simulink model "Assignment_2_RateAdaptive"  (R2020a)
settings: Solver=FixedStepAuto  StartTime=0.0  StopTime=10.0  FixedStep=1e-3  RelTol=1e-3  EnableMultiTasking=on
undefined symbols (not defined in the file): D0, D1, D10, D11, D12, D13, D2, D3, D4, D5, D6, D7, D8, D9, PTA0, PTA1, PTA2, PTB23, PTB9, PTC16, PTC17, PTC2, PTC3, PTC4, PTD0, PTD1, PTD2, PTD3
libraries: frdmk64flib x18, dspstat3 x1
settings Model: ExtModeTrigDuration=5  Creator=School  LastModifiedBy=logan_duui82v
settings OptimizationCC: EnhancedBackFolding=on  PassReuseOutputArgsAs=Individual arguments  ZeroExternalMemoryAtStartup=off  ZeroInternalMemoryAtStartup=off  MaxStackSize=64  OptimizeBlockOrder=speed  DifferentSizesBufferReuse=on  OptimizationCustomize=off  EfficientTunableParamExpr=on
settings DebuggingCC: ParameterTunabilityLossMsg=error
settings HardwareCC: ProdBitPerPointer=32  ProdBitPerSizeT=32  ProdBitPerPtrDiffT=32  ProdLargestAtomicInteger=Long  ProdLargestAtomicFloat=Double  ProdWordSize=32  ProdHWDeviceType=ARM Compatible->ARM Cortex
settings SFSimCC: MATLABDynamicMemAlloc=off
settings RTWCC: SystemTargetFile=ert.tlc  HardwareBoard=NXP FRDM-K64F  TemplateMakefile=ert_default_tmf  Toolchain=GNU Tools for ARM Embedded Processors
settings CodeAppCC: ForceParamTrailComments=on  IgnoreCustomStorageClasses=off  OperatorAnnotations=on  SimulinkDataObjDesc=on  SFDataObjDesc=on  InsertBlockDesc=on

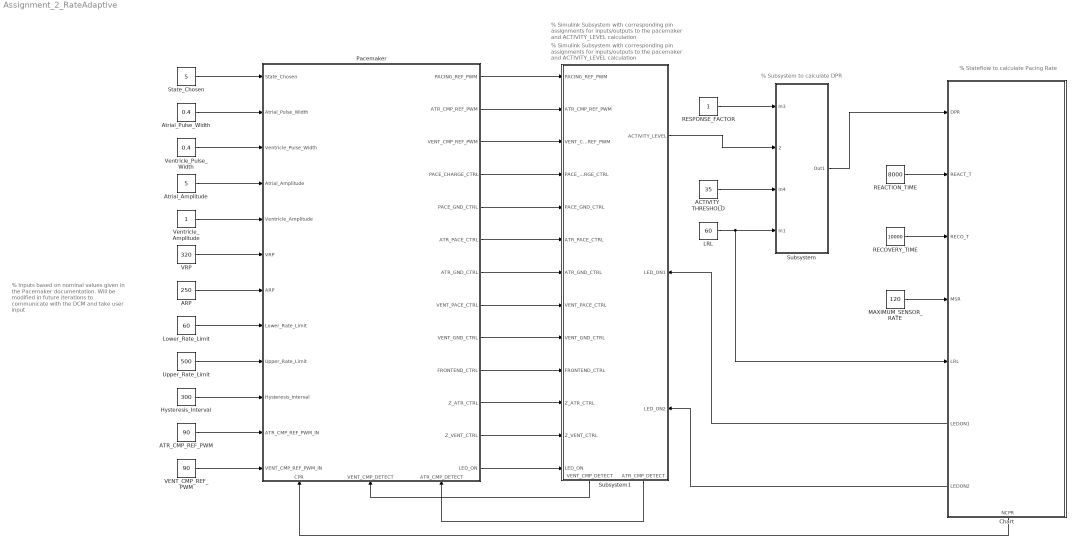
== system Assignment_2_RateAdaptive ==
  note: % Stateflow to calculate Pacing Rate
  note: % Inputs based on nominal values
      | given in the Pacemaker documentation.
      | Will be modified in future iterations to
      | communicate with the DCM and take
      | user input
  note: % Simulink Subsystem with corresponding pin
      | assignments for inputs/outputs to the pacemaker
      | and ACTIVITY_LEVEL calculation
  note: % Subsystem to calculate DPR
  note: % Simulink Subsystem with corresponding pin
      | assignments for inputs/outputs to the pacemaker
      | and ACTIVITY_LEVEL calculation
  ACTIVITY_THRESHOLD : Constant  Value=35
  ARP : Constant  Value=250
  ATR_CMP_REF_PWM : Constant  Value=90
  Atrial_Amplitude : Constant  Value=5  OutDataTypeStr=double
  Atrial_Pulse_Width : Constant  Value=0.4  OutDataTypeStr=int32
  Chart : Stateflow chart  TreatAsAtomicUnit=on
      settings: PortSchema="{\"entries\":[{\"content\":{\"sides\":[{\"content\":{\"connectorIds\":[\"In5\",\"In1\",\"In2\",\"In3\",\"In4\",\"Out2\",\"Out3\"]},\"type\":\"ConnectorPlacement.EquallySpacedRectSide\",\"uuid\":\"cb49ebd1-b2c7-4a1e-b062-18a1bf51e97f\"},{\"content\":{\"connectorIds\":[],\"side\":\"RIGHT\"},\"type\":\"ConnectorPlacement.EquallySpacedRectSide\",\"uuid\":\"35cf40a1-f02a-4965-9a15-2487395dd71b\"},{\"content\":{\"connectorIds\":[],\"side\":\"TOP\"},\"type\":\"ConnectorPlacement.EquallySpacedRectSide\",\"uuid\":\"8cf7664f-bebd-444c-a693-a1ee33fcaf3f\"},{\"content\":{\"connectorIds\":[\"Out1\"],\"side\":\"BOTTOM\"},\"type\":\"ConnectorPlacement.EquallySpacedRectSide\",\"uuid\":\"96b9c03b-a83e-462b-a12d-192e0bec7514\"}]},\"type\":\"ConnectorPlacement.EquallySpacedConnector\",\"uuid\":\"1030b27a-8fcd-482c-adda-aee1bfc69e16\"}],\"packageUris\":[\"http://schema.mathworks.com/mf0/Connector/19700101\"],\"version\":\"1.0\"}"
  Hysteresis_Interval : Constant  Value=300  OutDataTypeStr=int32
  LRL : Constant  Value=60
  Lower_Rate_Limit : Constant  Value=60  OutDataTypeStr=int32
  MAXIMUM_SENSOR_RATE : Constant  Value=120  OutDataTypeStr=double
  Pacemaker : Stateflow chart  TreatAsAtomicUnit=on
      settings: PortSchema="{\"entries\":[{\"content\":{\"sides\":[{\"content\":{\"connectorIds\":[\"In3\",\"In2\",\"In6\",\"In11\",\"In14\",\"In9\",\"In10\",\"In1\",\"In4\",\"In8\",\"In12\",\"In13\"]},\"type\":\"ConnectorPlacement.EquallySpacedRectSide\",\"uuid\":\"df877ca0-8245-4163-8fee-7182eab1d55d\"},{\"content\":{\"connectorIds\":[\"Out11\",\"Out12\",\"Out13\",\"Out2\",\"Out3\",\"Out1\",\"Out5\",\"Out7\",\"Out8\",\"Out10\",\"Out4\",\"Out9\",\"Out6\"],\"side\":\"RIGHT\"},\"type\":\"ConnectorPlacement.EquallySpacedRectSide\",\"uuid\":\"3a694184-6a85-4729-834f-a3ab7480664d\"},{\"content\":{\"connectorIds\":[],\"side\":\"TOP\"},\"type\":\"ConnectorPlacement.EquallySpacedRectSide\",\"uuid\":\"45b3d390-d3d3-4e22-8b52-b1590054c23a\"},{\"content\":{\"connectorIds\":[\"In15\",\"In7\",\"In5\"],\"side\":\"BOTTOM\"},\"type\":\"ConnectorPlacement.EquallySpacedRectSide\",\"uuid\":\"6c9e5202-d251-45f4-8fc3-f7acec5b4ccb\"}]},\"type\":\"ConnectorPlacement.EquallySpacedConnector\",\"uuid\":\"ad3b7ed4-c882-4247-8e15-d6beb1b6e9a6\"}],\"packageUris\":[\"http://schema.mathworks.com/mf0/Connector/19700101\"],\"version\":\"1.0\"}"
  REACTION_TIME : Constant  Value=8000  OutDataTypeStr=double
  RECOVERY_TIME : Constant  Value=10000  OutDataTypeStr=double
  RESPONSE_FACTOR : Constant
  State_Chosen : Constant  Value=5  OutDataTypeStr=int32
  Subsystem : Subsystem
  Subsystem1 : Subsystem
      settings: PortSchema="{\"entries\":[{\"content\":{\"sides\":[{\"content\":{\"connectorIds\":[\"In1\",\"In2\",\"In3\",\"In4\",\"In5\",\"In6\",\"In7\",\"In8\",\"In9\",\"In10\",\"In11\",\"In12\",\"In13\"]},\"type\":\"ConnectorPlacement.EquallySpacedRectSide\",\"uuid\":\"ef2db809-6ccb-4e10-b58a-4485458e2964\"},{\"content\":{\"connectorIds\":[\"Out1\",\"In14\",\"In15\"],\"side\":\"RIGHT\"},\"type\":\"ConnectorPlacement.EquallySpacedRectSide\",\"uuid\":\"23d27200-782c-4f65-a16b-b3dd9656ca92\"},{\"content\":{\"connectorIds\":[],\"side\":\"TOP\"},\"type\":\"ConnectorPlacement.EquallySpacedRectSide\",\"uuid\":\"4b957b3e-d3aa-4134-aa93-5dbe3bbb3ed9\"},{\"content\":{\"connectorIds\":[\"Out2\",\"Out3\"],\"side\":\"BOTTOM\"},\"type\":\"ConnectorPlacement.EquallySpacedRectSide\",\"uuid\":\"a8c808a9-b56b-4501-9a7a-854e8bc467f3\"}]},\"type\":\"ConnectorPlacement.EquallySpacedConnector\",\"uuid\":\"df464ebb-01b6-42d4-a9ed-9d5a529b4182\"}],\"packageUris\":[\"http://schema.mathworks.com/mf0/Connector/19700101\"],\"version\":\"1.0\"}"
  Upper_Rate_Limit : Constant  Value=500  OutDataTypeStr=int32
  VENT_CMP_REF_PWM : Constant  Value=90
  VRP : Constant  Value=320
  Ventricle_Amplitude : Constant
  Ventricle_Pulse_Width : Constant  Value=0.4  OutDataTypeStr=int32
  wires:
  Pacemaker/2(PACE_CHARGE_CTRL) -> Subsystem1/4(PACE_CHARGE_CTRL)
  Hysteresis_Interval/1 -> Pacemaker/8(Hysteresis_Interval)
  Chart/1(NCPR) -> Pacemaker/15(CPR)
  Chart/2(LEDON1) -> Subsystem1/14(LED_ON1)
  Pacemaker/7(VENT_PACE_CTRL) -> Subsystem1/8(VENT_PACE_CTRL)
  Chart/3(LEDON2) -> Subsystem1/15(LED_ON2)
  Ventricle_Amplitude/1 -> Pacemaker/14(Ventricle_Amplitude)
  Pacemaker/6(LED_ON) -> Subsystem1/13(LED_ON)
  VRP/1 -> Pacemaker/9(VRP)
  State_Chosen/1 -> Pacemaker/3(State_Chosen)
  Pacemaker/9(Z_VENT_CTRL) -> Subsystem1/12(Z_VENT_CTRL)
  REACTION_TIME/1 -> Chart/1(REACT_T)
  ACTIVITY_THRESHOLD/1 -> Subsystem/3(In4)
  RECOVERY_TIME/1 -> Chart/2(RECO_T)
  Pacemaker/10(FRONTEND_CTRL) -> Subsystem1/10(FRONTEND_CTRL)
  ARP/1 -> Pacemaker/10(ARP)
  Pacemaker/12(ATR_CMP_REF_PWM) -> Subsystem1/2(ATR_CMP_REF_PWM)
  Pacemaker/11(PACING_REF_PWM) -> Subsystem1/1(PACING_REF_PWM)
  ATR_CMP_REF_PWM/1 -> Pacemaker/12(ATR_CMP_REF_PWM_IN)
  Pacemaker/13(VENT_CMP_REF_PWM) -> Subsystem1/3(VENT_CMP_REF_PWM)
  MAXIMUM_SENSOR_RATE/1 -> Chart/3(MSR)
  Pacemaker/5(ATR_GND_CTRL) -> Subsystem1/7(ATR_GND_CTRL)
  Pacemaker/1(ATR_PACE_CTRL) -> Subsystem1/6(ATR_PACE_CTRL)
  VENT_CMP_REF_PWM/1 -> Pacemaker/13(VENT_CMP_REF_PWM_IN)
  Pacemaker/8(VENT_GND_CTRL) -> Subsystem1/9(VENT_GND_CTRL)
  Ventricle_Pulse_Width/1 -> Pacemaker/6(Ventricle_Pulse_Width)
  Subsystem/1(Out1) -> Chart/5(DPR)
  Pacemaker/3(PACE_GND_CTRL) -> Subsystem1/5(PACE_GND_CTRL)
  Subsystem1/2(" VENT_CMP_DETECT") -> Pacemaker/7(VENT_CMP_DETECT)
  Atrial_Pulse_Width/1 -> Pacemaker/2(Atrial_Pulse_Width)
  Atrial_Amplitude/1 -> Pacemaker/11(Atrial_Amplitude)
  Upper_Rate_Limit/1 -> Pacemaker/4(Upper_Rate_Limit)
  Pacemaker/4(Z_ATR_CTRL) -> Subsystem1/11(Z_ATR_CTRL)
  Subsystem1/3(ATR_CMP_DETECT) -> Pacemaker/5(ATR_CMP_DETECT)
  Lower_Rate_Limit/1 -> Pacemaker/1(Lower_Rate_Limit)
  LRL/1 -> Chart/4(LRL), Subsystem/4(In1)
  RESPONSE_FACTOR/1 -> Subsystem/1(In3)
  Subsystem1/1(ACTIVITY_LEVEL) -> Subsystem/2(2)

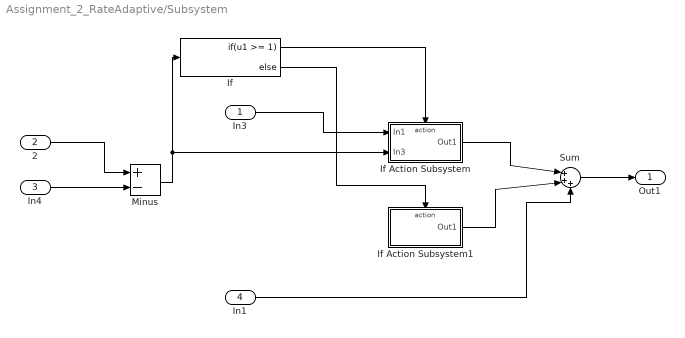
== system Assignment_2_RateAdaptive/Subsystem ==
  In3 : Inport
  2 : Inport  Port=2
  In4 : Inport  Port=3
  In1 : Inport  Port=4
  If : If  IfExpression=u1 >= 1
  If Action Subsystem : Subsystem  TreatAsAtomicUnit=on
  If Action Subsystem1 : Subsystem  TreatAsAtomicUnit=on
  Minus : Sum  Inputs=+-
  Sum : Sum  Inputs=|+++
  Out1 : Outport
  wires:
  2/1 -> Minus/1
  In4/1 -> Minus/2
  Minus/1 -> If Action Subsystem/2(In3), If/1
  If/1 -> If Action Subsystem/Action
  If/2 -> If Action Subsystem1/Action
  In3/1 -> If Action Subsystem/1(In1)
  Sum/1 -> Out1/1
  In1/1 -> Sum/3
  If Action Subsystem1/1(Out1) -> Sum/2
  If Action Subsystem/1(Out1) -> Sum/1

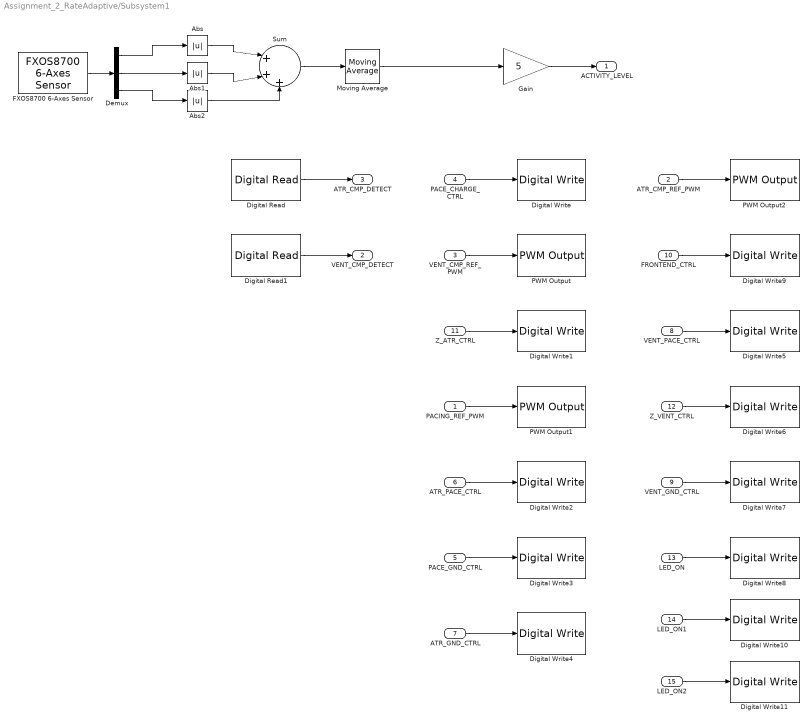
== system Assignment_2_RateAdaptive/Subsystem1 ==
  PACING_REF_PWM : Inport
  ATR_CMP_REF_PWM : Inport  Port=2
  VENT_CMP_REF_PWM : Inport  Port=3
  PACE_CHARGE_CTRL : Inport  Port=4
  PACE_GND_CTRL : Inport  Port=5
  ATR_PACE_CTRL : Inport  Port=6
  ATR_GND_CTRL : Inport  Port=7
  VENT_PACE_CTRL : Inport  Port=8
  VENT_GND_CTRL : Inport  Port=9
  FRONTEND_CTRL : Inport  Port=10
  Z_ATR_CTRL : Inport  Port=11
  Z_VENT_CTRL : Inport  Port=12
  LED_ON : Inport  Port=13
  LED_ON1 : Inport  Port=14
  LED_ON2 : Inport  Port=15
  Abs : Abs
  Abs1 : Abs
  Abs2 : Abs
  Demux : Demux  Outputs=3
  Digital Read : frdmk64flib/Digital Read  Whichpin=PTC16 (D0)  SampleTime=-1
  Digital Read1 : frdmk64flib/Digital Read  Whichpin=PTC17 (D1)  SampleTime=-1
  Digital Write : frdmk64flib/Digital Write  Whichpin=PTB9 (D2)
  Digital Write1 : frdmk64flib/Digital Write  Whichpin=PTB23 (D4)
  Digital Write10 : frdmk64flib/Digital Write  Whichpin=GREEN_LED
  Digital Write11 : frdmk64flib/Digital Write  Whichpin=BLUE_LED
  Digital Write2 : frdmk64flib/Digital Write  Whichpin=PTA0 (D8)
  Digital Write3 : frdmk64flib/Digital Write  Whichpin=PTD0 (D10)
  Digital Write4 : frdmk64flib/Digital Write  Whichpin=PTD2 (D11)
  Digital Write5 : frdmk64flib/Digital Write  Whichpin=PTC4 (D9)
  Digital Write6 : frdmk64flib/Digital Write  Whichpin=PTC3 (D7)
  Digital Write7 : frdmk64flib/Digital Write  Whichpin=PTD3 (D12)
  Digital Write8 : frdmk64flib/Digital Write  Whichpin=RED_LED
  Digital Write9 : frdmk64flib/Digital Write  Whichpin=PTD1 (D13)
  FXOS8700 6-Axes Sensor : frdmk64flib/FXOS8700 6-Axes Sensor  Activesensor=Accelerometer only  ODR=800Hz  HybridODR=400Hz  Accelfullrange=-4g to +4g  SampleTime=-1
  Gain : Gain  Gain=5
  Moving Average : dspstat3/Moving Average  Method=Sliding window  ForgettingFactorPort=off  SpecifyWindowLength=on  WindowLength=800  ForgettingFactor=0.9  SimulateUsing=Code generation
  PWM Output : frdmk64flib/PWM Output  Whichpin=PTA1 (D3)  InitialFrequency=2000  InitialDutyCycle=100
  PWM Output1 : frdmk64flib/PWM Output  Whichpin=PTA2 (D5)  InitialFrequency=2000  InitialDutyCycle=50
  PWM Output2 : frdmk64flib/PWM Output  Whichpin=PTC2 (D6)  InitialFrequency=2000  InitialDutyCycle=100
  Sum : Sum  Inputs=|+++
  ACTIVITY_LEVEL : Outport
  " VENT_CMP_DETECT" : Outport  Port=2
  ATR_CMP_DETECT : Outport  Port=3
  wires:
  Digital Read/1 -> ATR_CMP_DETECT/1
  Digital Read1/1 -> " VENT_CMP_DETECT"/1
  PACE_CHARGE_CTRL/1 -> Digital Write/1
  VENT_CMP_REF_PWM/1 -> PWM Output/1
  Z_ATR_CTRL/1 -> Digital Write1/1
  PACING_REF_PWM/1 -> PWM Output1/1
  ATR_PACE_CTRL/1 -> Digital Write2/1
  PACE_GND_CTRL/1 -> Digital Write3/1
  ATR_GND_CTRL/1 -> Digital Write4/1
  VENT_PACE_CTRL/1 -> Digital Write5/1
  Z_VENT_CTRL/1 -> Digital Write6/1
  VENT_GND_CTRL/1 -> Digital Write7/1
  LED_ON/1 -> Digital Write8/1
  ATR_CMP_REF_PWM/1 -> PWM Output2/1
  FRONTEND_CTRL/1 -> Digital Write9/1
  FXOS8700 6-Axes Sensor/1 -> Demux/1
  Demux/1 -> Abs/1
  Abs/1 -> Sum/1
  Abs1/1 -> Sum/2
  Demux/2 -> Abs1/1
  Demux/3 -> Abs2/1
  Abs2/1 -> Sum/3
  Gain/1 -> ACTIVITY_LEVEL/1
  Moving Average/1 -> Gain/1
  LED_ON1/1 -> Digital Write10/1
  LED_ON2/1 -> Digital Write11/1
  Sum/1 -> Moving Average/1

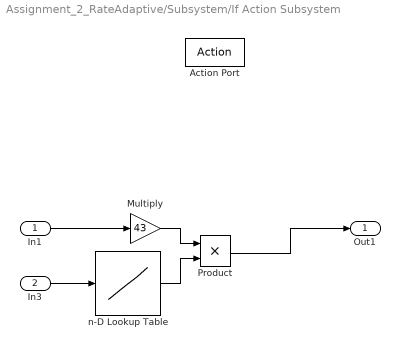
== system Assignment_2_RateAdaptive/Subsystem/If Action Subsystem ==
  In1 : Inport
  In3 : Inport  Port=2
  Action Port : ActionPort  ActionPortLabel=if(u1 >= 1)
  Multiply : Gain  Gain=43
  Product : Product  OutDataTypeStr=int8
  n-D Lookup Table : Lookup_n-D  NumberOfTableDimensions=1  LookupTableObject=log10  BreakpointsForDimension1=[1:55]  BreakpointsForDimension3=[5, 7]  Table="[0    0.3010    0.4771    0.6021    0.6990    0.7782    0.8451    0.9031    0.9542    1.0000    1.0414    1.0792    1.1139    1.1461    1.1761    1.2041    1.2304    1.2553    1.2788    1.3010    1.3222    1.3424    1.3617    1.3802    1.3979    1.4150    1.4314    1.4472    1.4624    1.4771    1.4914    1.5051    1.5185    1.5315    1.5441    1.5563    1.5682    1.5798    1.5911    1.6021    1.6128    1.6232    1.6335    1.6435    1.6532    1.6628    1.6721    1.6812    1.6902    1.6990    1.7076    1.7160    1.7243    1.7324    1.7404]"  InternalRulePriority=Speed  RndMeth=Simplest  InputSameDT=on
  Out1 : Outport
  wires:
  In1/1 -> Multiply/1
  In3/1 -> n-D Lookup Table/1
  Multiply/1 -> Product/1
  n-D Lookup Table/1 -> Product/2
  Product/1 -> Out1/1

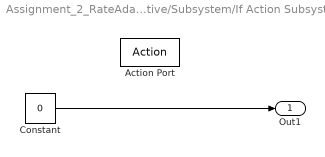
== system Assignment_2_RateAdaptive/Subsystem/If Action Subsystem1 ==
  Action Port : ActionPort  ActionPortLabel=else
  Constant : Constant  Value=0
  Out1 : Outport
  wires:
  Constant/1 -> Out1/1

== stateflow chart Assignment_2_RateAdaptive/Pacemaker ==
  settings: executeAtInitialization=1
  state AOO
    state ChargingDischarging
      entry:
      %No Sensing
      FRONTEND_CTRL = false;
      %Charging
      PACE_CHARGE_CTRL = true;
      ATR_PACE_CTRL = false;
      VENT_PACE_CTRL = false;
      PACING_REF_PWM = (Atrial_Amplitude/5) * 100;
      %Discharging
      PACE_GND_CTRL = true;
      ATR_PACE_CTRL = false;
      ATR_GND_CTRL = true;
      VENT_PACE_CTRL = false;
      VENT_GND_CTRL = false;
      Z_ATR_CTRL = false;
      Z_VENT_CTRL = false;
      LED_ON = false;
      LRL = 30000/Lower_Rate_Limit;
    state APacing
      entry:
      %Pace Atrial
      PACE_CHARGE_CTRL = false;
      PACE_GND_CTRL = true;
      ATR_PACE_CTRL = true;
      ATR_GND_CTRL = false;
      VENT_PACE_CTRL = false;
      VENT_GND_CTRL = false;
      Z_ATR_CTRL = false;
      Z_VENT_CTRL = false;
      LED_ON = true;
    note: % Charges until after the lower rate limit passes, sends a pulse for as long as the pulse width. Cycle repeats.
    (default) -> AOO.ChargingDischarging
    AOO.ChargingDischarging -> AOO.APacing : [after(LRL - Atrial_Pulse_Width, msec)]
    AOO.APacing -> AOO.ChargingDischarging : [after(Atrial_Pulse_Width,msec)]
  state VOO
    state ChargingDischarging
      entry:
      %No Sensing
      FRONTEND_CTRL = false;
      %Charging
      PACE_CHARGE_CTRL = true;
      ATR_PACE_CTRL = false;
      VENT_PACE_CTRL = false;
      PACING_REF_PWM = (Ventricle_Amplitude/5) * 100;
      %Discharging
      PACE_GND_CTRL = true;
      ATR_PACE_CTRL = false;
      ATR_GND_CTRL = false;
      VENT_PACE_CTRL = false;
      VENT_GND_CTRL = true;
      Z_ATR_CTRL = false;
      Z_VENT_CTRL = false;
      LED_ON = false;
      LRL = 30000/Lower_Rate_Limit;
    state VPacing
      entry:
      %Pace Ventricle
      PACE_CHARGE_CTRL = false;
      PACE_GND_CTRL = true;
      ATR_PACE_CTRL = false;
      ATR_GND_CTRL = false;
      VENT_PACE_CTRL = true;
      VENT_GND_CTRL = false;
      Z_ATR_CTRL = false;
      Z_VENT_CTRL = false;
      LED_ON = true;
    (default) -> VOO.ChargingDischarging
    VOO.ChargingDischarging -> VOO.VPacing : [after(LRL - Ventricle_Pulse_Width, msec)]
    VOO.VPacing -> VOO.ChargingDischarging : [after(Ventricle_Pulse_Width,msec)]
  state AAI
    state APacing
      entry:
      %Disable Sensing
      FRONTEND_CTRL = false;
      %Pace Atrial
      PACE_CHARGE_CTRL = false;
      PACE_GND_CTRL = true;
      ATR_PACE_CTRL = true;
      ATR_GND_CTRL = false;
      VENT_PACE_CTRL = false;
      VENT_GND_CTRL = false;
      Z_ATR_CTRL = false;
      Z_VENT_CTRL = false;
      LED_ON = true;
    state ChargingDischarging
      entry:
      %Enable Sensing
      FRONTEND_CTRL = true;
      ATR_CMP_REF_PWM = ATR_CMP_REF_PWM_IN
      %Charging
      PACE_CHARGE_CTRL = true;
      ATR_PACE_CTRL = false;
      VENT_PACE_CTRL = false;
      PACING_REF_PWM = (Atrial_Amplitude/5) * 100;
      %Discharging
      PACE_GND_CTRL = true;
      ATR_PACE_CTRL = false;
      ATR_GND_CTRL = true;
      VENT_PACE_CTRL = false;
      VENT_GND_CTRL = false;
      Z_ATR_CTRL = false;
      Z_VENT_CTRL = false;
      LED_ON = false;
      LRL = 30000/Lower_Rate_Limit;
    state Hysteresis
      entry:
      %Enable Sensing
      FRONTEND_CTRL = true;
      %Charging
      PACE_CHARGE_CTRL = true;
      ATR_PACE_CTRL = false;
      VENT_PACE_CTRL = false;
      %Discharging
      PACE_GND_CTRL = true;
      ATR_PACE_CTRL = false;
      ATR_GND_CTRL = true;
      VENT_PACE_CTRL = false;
      VENT_GND_CTRL = false;
      Z_ATR_CTRL = false;
      Z_VENT_CTRL = false;
      LED_ON = false;
    note: % If a natural heart beat is detected,
        | enter the Hysteresis state until no
        | natural beat occurs for the lower rate
        | limit plus the hysteresis interval
    (default) -> AAI.ChargingDischarging
    AAI.ChargingDischarging -> AAI.APacing [order 1] : [after(LRL - Atrial_Pulse_Width, msec)]
    AAI.APacing -> AAI.ChargingDischarging : [after(Atrial_Pulse_Width,msec)]
    AAI.Hysteresis -> AAI.APacing [order 1] : [after(LRL + Hysteresis_Interval, msec)]
    AAI.ChargingDischarging -> AAI.Hysteresis [order 2] : [after(ARP, msec) && ATR_CMP_DETECT == true]
    AAI.Hysteresis -> AAI.Hysteresis [order 2] : [after(ARP, msec) && ATR_CMP_DETECT == true]
  state VVI
    state ChargingDischarging
      entry:
      %Enable Sensing
      FRONTEND_CTRL = true;
      VENT_CMP_REF_PWM = VENT_CMP_REF_PWM_IN
      %Charging
      PACE_CHARGE_CTRL = true;
      ATR_PACE_CTRL = false;
      VENT_PACE_CTRL = false;
      PACING_REF_PWM = (Ventricle_Amplitude/5) * 100;
      %Discharging
      PACE_GND_CTRL = true;
      ATR_PACE_CTRL = false;
      ATR_GND_CTRL = false;
      VENT_PACE_CTRL = false;
      VENT_GND_CTRL = true;
      Z_ATR_CTRL = false;
      Z_VENT_CTRL = false;
      LED_ON = false;
      LRL = 30000/Lower_Rate_Limit;
    state VPacing
      entry:
      %Disable Sensing
      FRONTEND_CTRL = false;
      %Pace Ventricle
      PACE_CHARGE_CTRL = false;
      PACE_GND_CTRL = true;
      ATR_PACE_CTRL = false;
      ATR_GND_CTRL = false;
      VENT_PACE_CTRL = true;
      VENT_GND_CTRL = false;
      Z_ATR_CTRL = false;
      Z_VENT_CTRL = false;
      LED_ON = true;
    state Hysteresis
      entry:
      %Enable Sensing
      FRONTEND_CTRL = true;
      %Charging
      PACE_CHARGE_CTRL = true;
      ATR_PACE_CTRL = false;
      VENT_PACE_CTRL = false;
      %Discharging
      PACE_GND_CTRL = true;
      ATR_PACE_CTRL = false;
      ATR_GND_CTRL = false;
      VENT_PACE_CTRL = false;
      VENT_GND_CTRL = true;
      Z_ATR_CTRL = false;
      Z_VENT_CTRL = false;
      LED_ON = false;
    (default) -> VVI.ChargingDischarging
    VVI.ChargingDischarging -> VVI.VPacing [order 1] : [after(LRL - Ventricle_Pulse_Width, msec)]
    VVI.VPacing -> VVI.ChargingDischarging : [after(Ventricle_Pulse_Width,msec)]
    VVI.Hysteresis -> VVI.VPacing [order 2] : [after(LRL + Hysteresis_Interval, msec)]
    VVI.ChargingDischarging -> VVI.Hysteresis [order 2] : [after(VRP, msec) && VENT_CMP_DETECT==true]
    VVI.Hysteresis -> VVI.Hysteresis [order 1] : [after(VRP, msec) && VENT_CMP_DETECT==true]
  state initialState
  note: % Upon startup, pacemaker goes into the selected
      | mode based on the "State_Chosen" variable
  state AOOR
    state ChargingDischarging
      entry:
      %No Sensing
      FRONTEND_CTRL = false;
      %Charging
      PACE_CHARGE_CTRL = true;
      ATR_PACE_CTRL = false;
      VENT_PACE_CTRL = false;
      PACING_REF_PWM = (Atrial_Amplitude/5) * 100;
      %Discharging
      PACE_GND_CTRL = true;
      ATR_PACE_CTRL = false;
      ATR_GND_CTRL = true;
      VENT_PACE_CTRL = false;
      VENT_GND_CTRL = false;
      Z_ATR_CTRL = false;
      Z_VENT_CTRL = false;
      LED_ON = false;
      PACE = 30000/CPR;
    state APacing
      entry:
      %Pace Atrial
      PACE_CHARGE_CTRL = false;
      PACE_GND_CTRL = true;
      ATR_PACE_CTRL = true;
      ATR_GND_CTRL = false;
      VENT_PACE_CTRL = false;
      VENT_GND_CTRL = false;
      Z_ATR_CTRL = false;
      Z_VENT_CTRL = false;
      LED_ON = true;
    note: % Charges until after the lower rate limit passes, sends a pulse for as long as the pulse width. Cycle repeats.
    (default) -> AOOR.ChargingDischarging
    AOOR.ChargingDischarging -> AOOR.APacing : [after(PACE - Atrial_Pulse_Width, msec)]
    AOOR.APacing -> AOOR.ChargingDischarging : [after(Atrial_Pulse_Width,msec)]
  state VOOR
    state ChargingDischarging
      entry:
      %No Sensing
      FRONTEND_CTRL = false;
      %Charging
      PACE_CHARGE_CTRL = true;
      ATR_PACE_CTRL = false;
      VENT_PACE_CTRL = false;
      PACING_REF_PWM = (Ventricle_Amplitude/5) * 100;
      %Discharging
      PACE_GND_CTRL = true;
      ATR_PACE_CTRL = false;
      ATR_GND_CTRL = false;
      VENT_PACE_CTRL = false;
      VENT_GND_CTRL = true;
      Z_ATR_CTRL = false;
      Z_VENT_CTRL = false;
      LED_ON = false;
      PACE = 30000/CPR;
    state VPacing
      entry:
      %Pace Ventricle
      PACE_CHARGE_CTRL = false;
      PACE_GND_CTRL = true;
      ATR_PACE_CTRL = false;
      ATR_GND_CTRL = false;
      VENT_PACE_CTRL = true;
      VENT_GND_CTRL = false;
      Z_ATR_CTRL = false;
      Z_VENT_CTRL = false;
      LED_ON = true;
    (default) -> VOOR.ChargingDischarging
    VOOR.ChargingDischarging -> VOOR.VPacing : [after(PACE - Ventricle_Pulse_Width, msec)]
    VOOR.VPacing -> VOOR.ChargingDischarging : [after(Ventricle_Pulse_Width,msec)]
  state AAIR
    state APacing
      entry:
      %Disable Sensing
      FRONTEND_CTRL = false;
      %Pace Atrial
      PACE_CHARGE_CTRL = false;
      PACE_GND_CTRL = true;
      ATR_PACE_CTRL = true;
      ATR_GND_CTRL = false;
      VENT_PACE_CTRL = false;
      VENT_GND_CTRL = false;
      Z_ATR_CTRL = false;
      Z_VENT_CTRL = false;
      LED_ON = true;
    state ChargingDischarging
      entry:
      %Enable Sensing
      FRONTEND_CTRL = true;
      ATR_CMP_REF_PWM = ATR_CMP_REF_PWM_IN
      %Charging
      PACE_CHARGE_CTRL = true;
      ATR_PACE_CTRL = false;
      VENT_PACE_CTRL = false;
      PACING_REF_PWM = (Atrial_Amplitude/5) * 100;
      %Discharging
      PACE_GND_CTRL = true;
      ATR_PACE_CTRL = false;
      ATR_GND_CTRL = true;
      VENT_PACE_CTRL = false;
      VENT_GND_CTRL = false;
      Z_ATR_CTRL = false;
      Z_VENT_CTRL = false;
      LED_ON = false;
      PACE = 30000/CPR;
    state Hysteresis
      entry:
      %Enable Sensing
      FRONTEND_CTRL = true;
      %Charging
      PACE_CHARGE_CTRL = true;
      ATR_PACE_CTRL = false;
      VENT_PACE_CTRL = false;
      %Discharging
      PACE_GND_CTRL = true;
      ATR_PACE_CTRL = false;
      ATR_GND_CTRL = true;
      VENT_PACE_CTRL = false;
      VENT_GND_CTRL = false;
      Z_ATR_CTRL = false;
      Z_VENT_CTRL = false;
      LED_ON = false;
    note: % If a natural heart beat is detected,
        | enter the Hysteresis state until no
        | natural beat occurs for the lower rate
        | limit plus the hysteresis interval
    (default) -> AAIR.ChargingDischarging
    AAIR.ChargingDischarging -> AAIR.APacing [order 1] : [after(PACE - Atrial_Pulse_Width, msec)]
    AAIR.APacing -> AAIR.ChargingDischarging : [after(Atrial_Pulse_Width,msec)]
    AAIR.Hysteresis -> AAIR.APacing [order 1] : [after(PACE + Hysteresis_Interval, msec)]
    AAIR.ChargingDischarging -> AAIR.Hysteresis [order 2] : [after(ARP, msec) && ATR_CMP_DETECT == true]
    AAIR.Hysteresis -> AAIR.Hysteresis [order 2] : [after(ARP, msec) && ATR_CMP_DETECT == true]
  state VVIR
    state ChargingDischarging
      entry:
      %Enable Sensing
      FRONTEND_CTRL = true;
      VENT_CMP_REF_PWM = VENT_CMP_REF_PWM_IN
      %Charging
      PACE_CHARGE_CTRL = true;
      ATR_PACE_CTRL = false;
      VENT_PACE_CTRL = false;
      PACING_REF_PWM = (Ventricle_Amplitude/5) * 100;
      %Discharging
      PACE_GND_CTRL = true;
      ATR_PACE_CTRL = false;
      ATR_GND_CTRL = false;
      VENT_PACE_CTRL = false;
      VENT_GND_CTRL = true;
      Z_ATR_CTRL = false;
      Z_VENT_CTRL = false;
      LED_ON = false;
      PACE = 30000/CPR;
    state VPacing
      entry:
      %Disable Sensing
      FRONTEND_CTRL = false;
      %Pace Ventricle
      PACE_CHARGE_CTRL = false;
      PACE_GND_CTRL = true;
      ATR_PACE_CTRL = false;
      ATR_GND_CTRL = false;
      VENT_PACE_CTRL = true;
      VENT_GND_CTRL = false;
      Z_ATR_CTRL = false;
      Z_VENT_CTRL = false;
      LED_ON = true;
    state Hysteresis
      entry:
      %Enable Sensing
      FRONTEND_CTRL = true;
      %Charging
      PACE_CHARGE_CTRL = true;
      ATR_PACE_CTRL = false;
      VENT_PACE_CTRL = false;
      %Discharging
      PACE_GND_CTRL = true;
      ATR_PACE_CTRL = false;
      ATR_GND_CTRL = false;
      VENT_PACE_CTRL = false;
      VENT_GND_CTRL = true;
      Z_ATR_CTRL = false;
      Z_VENT_CTRL = false;
      LED_ON = false;
    (default) -> VVIR.ChargingDischarging
    VVIR.ChargingDischarging -> VVIR.VPacing [order 1] : [after(PACE - Ventricle_Pulse_Width, msec)]
    VVIR.VPacing -> VVIR.ChargingDischarging : [after(Ventricle_Pulse_Width,msec)]
    VVIR.Hysteresis -> VVIR.VPacing : [after(PACE + Hysteresis_Interval, msec)]
    VVIR.ChargingDischarging -> VVIR.Hysteresis [order 2] : [after(VRP, msec) && VENT_CMP_DETECT==true]
  initialState -> AOO [order 1] : [State_Chosen==1]
  initialState -> VOO [order 2] : [State_Chosen==2]
  initialState -> AAI [order 3] : [State_Chosen==3]
  initialState -> VVI [order 4] : [State_Chosen==4]
  (default) -> initialState
  initialState -> AOOR [order 8] : [State_Chosen==5]
  initialState -> VOOR [order 5] : [State_Chosen==6]
  initialState -> AAIR [order 6] : [State_Chosen==7]
  initialState -> VVIR [order 7] : [State_Chosen==8]
  data: Lower_Rate_Limit input int32; Atrial_Pulse_Width input int32; State_Chosen input int32; Upper_Rate_Limit input; ATR_PACE_CTRL output boolean =false; PACE_CHARGE_CTRL output boolean =false; PACE_GND_CTRL output boolean =false; Z_ATR_CTRL output boolean =false; ATR_GND_CTRL output boolean =false; LED_ON output boolean; VENT_PACE_CTRL output boolean; VENT_GND_CTRL output; Z_VENT_CTRL output; ATR_CMP_DETECT input boolean; Ventricle_Pulse_Width input int32; VENT_CMP_DETECT input; Hysteresis_Interval input int32; FRONTEND_CTRL output; VRP input; ARP input; PACING_REF_PWM output; ATR_CMP_REF_PWM output; VENT_CMP_REF_PWM output; Atrial_Amplitude input; ATR_CMP_REF_PWM_IN input; VENT_CMP_REF_PWM_IN input; Ventricle_Amplitude input; CPR input; LRL local; PACE local

== stateflow chart Assignment_2_RateAdaptive/Chart ==
  state State1
    entry:
    NCPR = 60;
  state Increasing
    entry:
    ROC = (MSR-LRL)/REACT_T;
    if NCPR > MSR
    NCPR = MSR;
    elseif NCPR <= LRL
    NCPR = LRL;
    elseif NCPR >= DPR
    NCPR = DPR;
    end
    LEDON1 = true;
    LEDON2 = false;
  state Decreasing
    entry:
    ROC = (MSR-LRL)/RECO_T;
    if NCPR <= LRL
    NCPR = LRL;
    elseif NCPR > MSR
    NCPR = MSR;
    elseif NCPR <= DPR
    NCPR = DPR;
    end
    LEDON1 = false;
    LEDON2 = true;
  (default) -> State1
  State1 -> Decreasing : [after(10, msec)]
  Decreasing -> Increasing [order 1] : [DPR > NCPR]
  Decreasing -> Decreasing [order 2] : [after(1, msec)]{NCPR = NCPR - ROC}
  Increasing -> Increasing [order 2] : [after(1, msec)]{NCPR = NCPR + ROC}
  Increasing -> Decreasing [order 1] : [DPR < NCPR]
  data: REACT_T input double; RECO_T input double; MSR input double; LRL input double; NCPR output double; DPR input; LEDON1 output; LEDON2 output; ROC local
